simulink model "twoUpDownCnts"  (R2025b)
settings: Solver=FixedStepDiscrete  StartTime=0.0  StopTime=Inf  RelTol=1e-3
settings Model: Creator=Soochan Kim  LastModifiedBy=Soochan Kim
settings OptimizationCC: BlockReduction=off  ConditionallyExecuteInputs=off  DefaultParameterBehavior=Inlined
settings DebuggingCC: AlgebraicLoopMsg=error
settings HardwareCC: ProdBitPerPointer=32.0  ProdBitPerSizeT=32.0  ProdBitPerPtrDiffT=32.0  ProdLargestAtomicFloat=None  ProdIntDivRoundTo=Undefined  ProdEndianess=Unspecified  ProdWordSize=32.0  ProdHWDeviceType=ASIC/FPGA->ASIC/FPGA  TargetBitPerPointer=64.0  TargetBitPerSizeT=64.0  TargetBitPerPtrDiffT=64.0  TargetLongLongMode=on  TargetIntDivRoundTo=Zero  TargetEndianess=LittleEndian  TargetWordSize=64.0  TargetHWDeviceType=Custom Processor->MATLAB Host Computer  ProdEqTarget=off

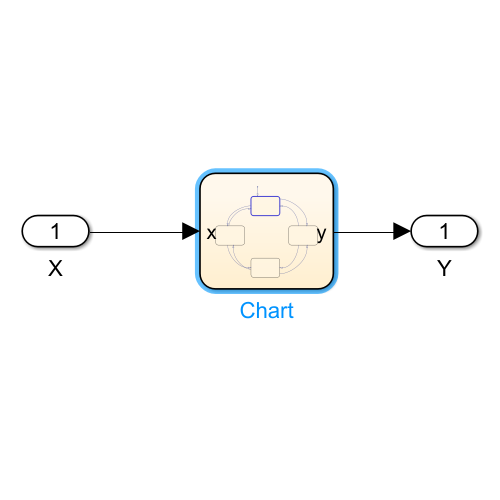
[thumbnail: Simulink's stored preview of the top-level diagram]
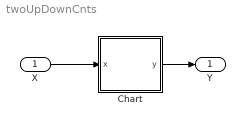
== system twoUpDownCnts ==
  X : Inport  OutDataTypeStr=boolean
  Chart : Stateflow chart  TreatAsAtomicUnit=on
  Y : Outport
  wires:
  X/1 -> Chart/1(x)
  Chart/1(y) -> Y/1

== stateflow chart twoUpDownCnts/Chart ==
  settings: updateMethod=DISCRETE  stateMachineType=MOORE_MACHINE  executeAtInitialization=1  initializeOutput=1
  state S0
    y=uint8(0);
  state S1
    y=uint8(1);
  state S3
    y=uint8(3);
  state S2
    y=uint8(2);
  (default) -> S0
  S0 -> S3 [order 2] : [x==0]
  S3 -> S0 [order 1] : [x==1]
  S0 -> S1 [order 1] : [x==1]
  S1 -> S0 [order 2] : [x==0]
  S1 -> S2 [order 1] : [x==1]
  S2 -> S1 [order 2] : [x==0]
  S2 -> S3 [order 1] : [x==1]
  S3 -> S2 [order 2] : [x==0]
  data: x input boolean; y output uint8
